simulink model "msdDoubleSoln"  (R2020b)
settings: Solver=VariableStepAuto  StartTime=0.0  StopTime=20  RelTol=1e-6
settings Model: Creator=Rocksmithed  LastModifiedBy=Rocksmithed

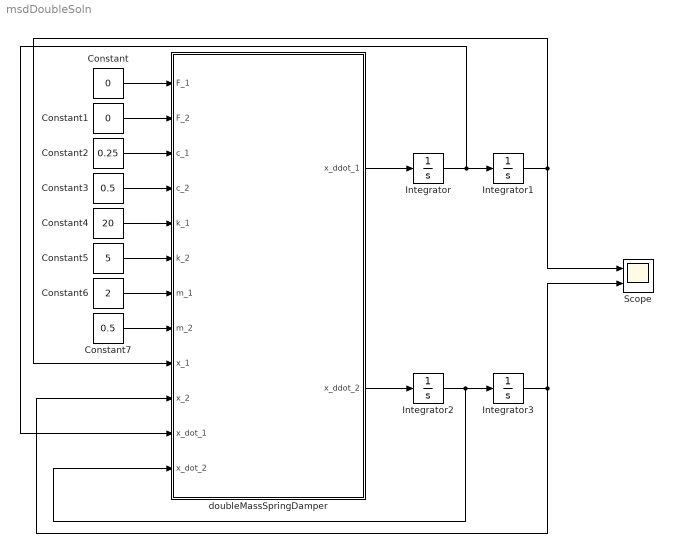
== system msdDoubleSoln ==
  Constant : Constant  Value=0
  Constant1 : Constant  Value=0
  Constant2 : Constant  Value=0.25
  Constant3 : Constant  Value=0.5
  Constant4 : Constant  Value=20
  Constant5 : Constant  Value=5
  Constant6 : Constant  Value=2
  Constant7 : Constant  Value=0.5
  Integrator : Integrator
  Integrator1 : Integrator
  Integrator2 : Integrator  InitialCondition=8
  Integrator3 : Integrator
  Scope : Scope  NumInputPorts=2
  doubleMassSpringDamper : MATLAB Function  TreatAsAtomicUnit=on
  wires:
  Constant/1 -> doubleMassSpringDamper/1(F_1)
  Constant1/1 -> doubleMassSpringDamper/2(F_2)
  Constant2/1 -> doubleMassSpringDamper/3(c_1)
  Constant3/1 -> doubleMassSpringDamper/4(c_2)
  Constant4/1 -> doubleMassSpringDamper/5(k_1)
  Constant5/1 -> doubleMassSpringDamper/6(k_2)
  Constant6/1 -> doubleMassSpringDamper/7(m_1)
  Constant7/1 -> doubleMassSpringDamper/8(m_2)
  doubleMassSpringDamper/1(x_ddot_1) -> Integrator/1
  Integrator/1 -> doubleMassSpringDamper/11(x_dot_1), Integrator1/1
  doubleMassSpringDamper/2(x_ddot_2) -> Integrator2/1
  Integrator2/1 -> doubleMassSpringDamper/12(x_dot_2), Integrator3/1
  Integrator1/1 -> doubleMassSpringDamper/9(x_1), Scope/1
  Integrator3/1 -> Scope/2, doubleMassSpringDamper/10(x_2)

== matlab function msdDoubleSoln/doubleMassSpringDamper ==
  data: F_1 input; x_ddot_1 output; F_2 input; c_1 input; c_2 input; k_1 input; k_2 input; m_1 input; m_2 input; x_1 input; x_2 input; x_dot_1 input; x_dot_2 input; x_ddot_2 output
function [x_ddot_1,x_ddot_2] = doubleMassSpringDamper(F_1,F_2,c_1,c_2,k_1,k_2,m_1,m_2,x_1,x_2,x_dot_1,x_dot_2)
%#codegen

%    This function was generated by the Symbolic Math Toolbox version 8.6.
%    19-Nov-2020 15:46:02

x_ddot_1 = -(-F_1+c_1.*x_dot_1+k_1.*x_1+c_2.*(x_dot_1-x_dot_2)+k_2.*(x_1-x_2))./m_1;
if nargout > 1
    x_ddot_2 = (F_2+c_2.*(x_dot_1-x_dot_2)+k_2.*(x_1-x_2))./m_2;
end
